simulink model "am_deslx"  (R2016a)
settings: Solver=VariableStepAuto  StartTime=0.0  StopTime=10.0  RelTol=1e-3
libraries: dsparch4 x1
settings Model: Creator=iP Store  LastModifiedBy=iP Store

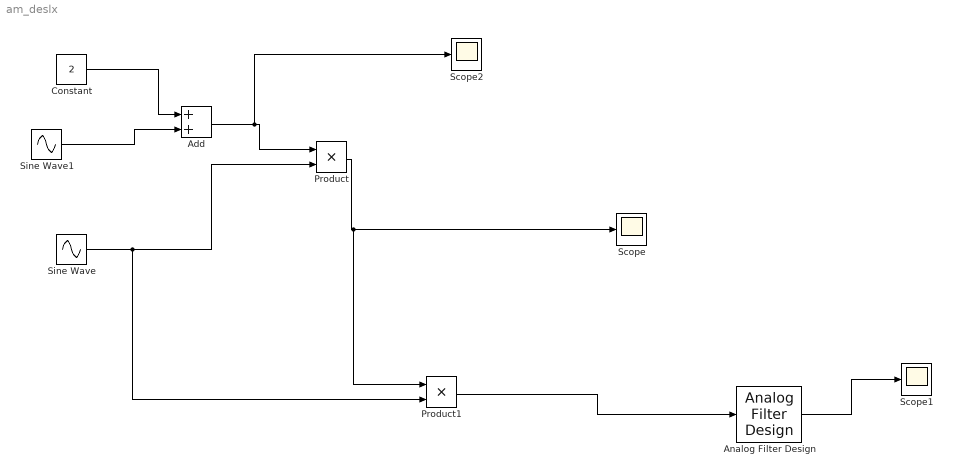
== system am_deslx ==
  Add : Sum
  Analog Filter Design : dsparch4/Analog Filter Design  method=Butterworth  filttype=Lowpass  N=8  Wlo=2e+3  Whi=80  Rp=2  Rs=40
  Constant : Constant  Value=2
  Product : Product
  Product1 : Product
  Scope : Scope
  Scope1 : Scope
  Scope2 : Scope
  Sine Wave : Sin  Frequency=100e+3  SampleTime=0
  Sine Wave1 : Sin  Frequency=2e+3  Phase=-pi/2  SampleTime=0
  wires:
  Sine Wave1/1 -> Add/2
  Constant/1 -> Add/1
  Add/1 -> Scope2/1, Product/1
  Product/1 -> Product1/1, Scope/1
  Sine Wave/1 -> Product1/2, Product/2
  Product1/1 -> Analog Filter Design/1
  Analog Filter Design/1 -> Scope1/1
